simulink model "SSBSC"  (R2023b)
settings: Solver=VariableStepAuto  StartTime=0.0  StopTime=20  RelTol=1e-3
libraries: commutil2 x1, commanapbnd3 x1, simulink x1
settings Model: Creator=HP  LastModifiedBy=HP

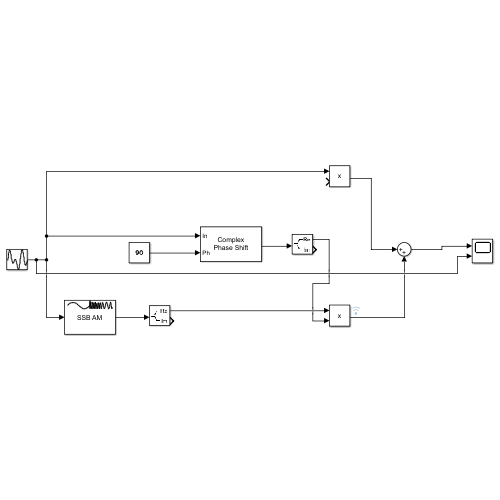
[thumbnail: Simulink's stored preview of the top-level diagram]
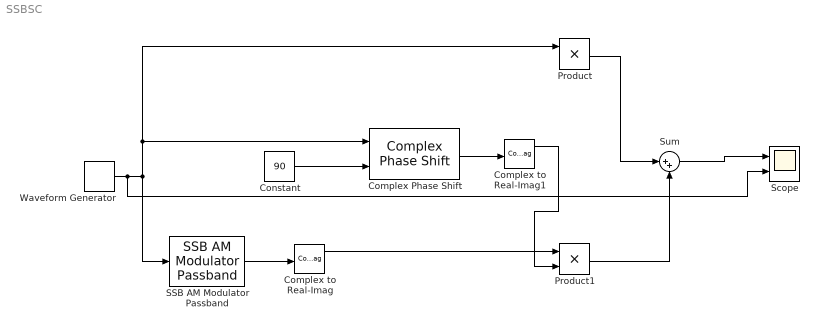
== system SSBSC ==
  Complex Phase Shift : commutil2/Complex Phase Shift
  Complex to Real-Imag : ComplexToRealImag
  Complex to Real-Imag1 : ComplexToRealImag
  Constant : Constant  Value=90
  Product : Product
  Product1 : Product
  SSB AM Modulator Passband : commanapbnd3/SSB AM Modulator Passband  Fc=300  Ph=0  Sd=Upper  Ho=100
  Scope : Scope  NumInputPorts=2
  Sum : Sum  Inputs=|++
  Waveform Generator : simulink/Sources/Waveform Generator  OutMin=[]  OutMax=[]  OutDataTypeStr=double  SelectedSignal=1  Signals=sin(5,10,1)  BlockNames=MultiportSwitch_2349eaff455e474  SampleTime=0.1
  wires:
  Waveform Generator/1 -> Scope/2, SSB AM Modulator Passband/1, Complex Phase Shift/1, Product/1
  SSB AM Modulator Passband/1 -> Complex to Real-Imag/1
  Complex to Real-Imag/1 -> Product1/1
  Constant/1 -> Complex Phase Shift/2
  Product/1 -> Sum/1
  Complex Phase Shift/1 -> Complex to Real-Imag1/1
  Complex to Real-Imag1/1 -> Product1/2
  Product1/1 -> Sum/2
  Sum/1 -> Scope/1
